simulink model "ThermalSystem2026 (3)"  (R2024b)
settings: Solver=VariableStepAuto  StartTime=0.0  StopTime=1296  RelTol=1e-3
settings Model: Creator=arthe  LastModifiedBy=arthe

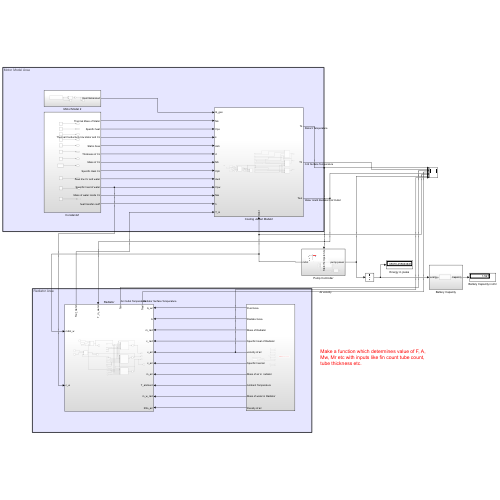
[thumbnail: Simulink's stored preview of the top-level diagram]
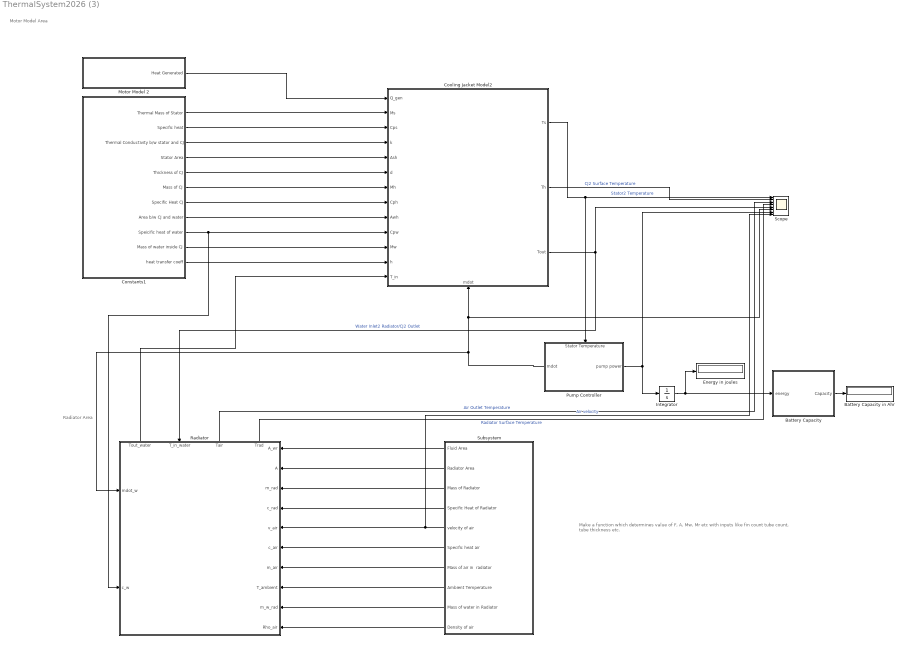
== system ThermalSystem2026 (3) ==
  note: Motor Model Area
  note: Radiator Area
  note: Make a function which determines value of F, A, Mw, Mr etc with inputs like fin count tube count, tube thickness etc.
  Battery Capacity : Subsystem
  Battery Capacity in Ahr : Display
  Constants1 : Subsystem
  Cooling Jacket Model2 : Subsystem
      settings: PortSchema="{\"entries\":[{\"content\":{\"sides\":[{\"content\":{\"connectorIds\":[\"In1\",\"In2\",\"In3\",\"In4\",\"In5\",\"In6\",\"In7\",\"In8\",\"In9\",\"In10\",\"In11\",\"In12\",\"In13\"]},\"type\":\"ConnectorPlacement.EquallySpacedRectSide\",\"uuid\":\"79d4d8e8-7803-45a2-afaa-4d22d6373157\"},{\"content\":{\"connectorIds\":[\"Out1\",\"Out2\",\"Out3\"],\"side\":\"RIGHT\"},\"type\":\"ConnectorPlacement.EquallySpacedRectSide\",\"uuid\":\"8eb2a985-3df9-4fca-ba99-d41949146ffd\"},{\"content\":{\"side\":\"TOP\"},\"type\":\"ConnectorPlacement.EquallySpacedRectSide\",\"uuid\":\"b6891a69-1971-4846-8973-0960fda02d22\"},{\"content\":{\"connectorIds\":[\"In14\"],\"side\":\"BOTTOM\"},\"type\":\"ConnectorPlacement.EquallySpacedRectSide\",\"uuid\":\"634c1221-39cf-4d03-a1b5-5507eb554710\"}]},\"type\":\"ConnectorPlacement.EquallySpacedConnector\",\"uuid\":\"d4f46766-14f9-4a8b-8c89-842668bdd4e0\"}],\"packageUris\":[\"http://schema.mathworks.com/mf0/Connector/R2020b\"],\"version\":\"1.0\"}"
  Energy in joules : Display
  Integrator : Integrator
  Motor Model 2 : Subsystem
  Pump Controller : Subsystem
      settings: PortSchema="{\"entries\":[{\"content\":{\"sides\":[{\"content\":{\"connectorIds\":[\"Out2\"]},\"type\":\"ConnectorPlacement.EquallySpacedRectSide\",\"uuid\":\"64509805-f0eb-407f-8df6-2012a67b9b8d\"},{\"content\":{\"connectorIds\":[\"Out1\"],\"side\":\"RIGHT\"},\"type\":\"ConnectorPlacement.EquallySpacedRectSide\",\"uuid\":\"85313de9-6d64-4d1e-8ebf-8c6fc6989453\"},{\"content\":{\"connectorIds\":[\"In1\"],\"side\":\"TOP\"},\"type\":\"ConnectorPlacement.EquallySpacedRectSide\",\"uuid\":\"4a1f9497-bef9-4f57-9d3c-2e3adca4de23\"}]},\"type\":\"ConnectorPlacement.EquallySpacedConnector\",\"uuid\":\"adca88aa-a89d-4531-9c32-6fc4488ac11c\"}],\"packageUris\":[\"http://schema.mathworks.com/mf0/Connector/R2020b\"],\"version\":\"1.0\"}"
  Radiator : Subsystem
      settings: PortSchema="{\"entries\":[{\"content\":{\"sides\":[{\"content\":{\"connectorIds\":[\"In1\",\"In2\",\"In3\",\"In4\",\"In5\",\"In6\",\"In7\",\"In8\",\"In9\",\"In10\"]},\"type\":\"ConnectorPlacement.EquallySpacedRectSide\",\"uuid\":\"442aa9ac-1748-45b5-b106-b2ea8ec9ba9a\"},{\"content\":{\"connectorIds\":[\"In12\",\"In13\"],\"side\":\"RIGHT\"},\"type\":\"ConnectorPlacement.EquallySpacedRectSide\",\"uuid\":\"346b8b1e-5690-410f-bffd-8882456125cf\"},{\"content\":{\"connectorIds\":[\"Out1\",\"Out2\",\"In11\",\"Out3\"],\"side\":\"TOP\"},\"type\":\"ConnectorPlacement.EquallySpacedRectSide\",\"uuid\":\"f47d136f-1f63-473a-b7aa-2f4bff6d0484\"}]},\"type\":\"ConnectorPlacement.EquallySpacedConnector\",\"uuid\":\"8ddbc53c-7178-458d-9bbd-f7e4bafa7e83\"}],\"packageUris\":[\"http://schema.mathworks.com/mf0/Connector/R2020b\"],\"version\":\"1.0\"}"
  Scope : Scope  NumInputPorts=8
  Subsystem : Subsystem
  wires:
  Constants1/7(Specific Heat CJ) -> Cooling Jacket Model2/8(Cph)
  Constants1/3(Thermal Conductivity b/w stator and CJ) -> Cooling Jacket Model2/4(k)
  Constants1/2(Specific heat) -> Cooling Jacket Model2/3(Cps)
  Constants1/11(heat transfer coeff) -> Cooling Jacket Model2/12(h)
  Constants1/10(Mass of water inside CJ) -> Cooling Jacket Model2/11(Mw)
  Constants1/8(Area b/w CJ and water) -> Cooling Jacket Model2/9(Awh)
  Constants1/5(Thickness of CJ) -> Cooling Jacket Model2/6(d)
  Constants1/1(Thermal Mass of Stator) -> Cooling Jacket Model2/2(Ms)
  Constants1/4(Stator Area) -> Cooling Jacket Model2/5(Ash)
  Constants1/6(Mass of CJ) -> Cooling Jacket Model2/7(Mh)
  Radiator/3(Tout_water) -> Cooling Jacket Model2/13(T_in)
  Cooling Jacket Model2/1(Ts) -> Scope/1, Pump Controller/1(Stator Temperature)  "Stator2 Temperature"
  Cooling Jacket Model2/2(Th) -> Scope/2  "CJ2 Surface Temperature"
  Cooling Jacket Model2/3(Tout) -> Radiator/11(T_in_water), Scope/5  "Water Inlet2 Radiator/CJ2 Outlet"
  Subsystem/8(Ambient Temperature) -> Radiator/8(T_ambient)
  Subsystem/3(Mass of Radiator) -> Radiator/3(m_rad)
  Subsystem/6(Specific heat air) -> Radiator/6(c_air)
  Subsystem/10(Density of air) -> Radiator/10(Rho_air)
  Subsystem/5(velocity of air) -> Scope/8, Radiator/5(v_air)  "Air velocity"
  Subsystem/4(Specific Heat of Radiator) -> Radiator/4(c_rad)
  Subsystem/7(Mass of air in  radiator) -> Radiator/7(m_air)
  Subsystem/9(Mass of water in Radiator) -> Radiator/9(m_w_rad)
  Subsystem/1("Fluid Area ") -> Radiator/1(A_wr)
  Subsystem/2(Radiator Area) -> Radiator/2(A)
  Radiator/1(Trad) -> Scope/4  "Radiator Surface Temperature"
  Radiator/2(Tair) -> Scope/3  "Air Outlet Temperature"
  Constants1/9(Speicific heat of water) -> Radiator/13(c_w), Cooling Jacket Model2/10(Cpw)
  Pump Controller/2(mdot) -> Radiator/12(mdot_w), Cooling Jacket Model2/14(mdot), Scope/6
  Pump Controller/1(pump power) -> Integrator/1, Scope/7
  Motor Model 2/1(Heat Generated) -> Cooling Jacket Model2/1(Q_gen)
  Integrator/1 -> Battery Capacity/1(energy), Energy in joules/1
  Battery Capacity/1(Capacity) -> Battery Capacity in Ahr/1

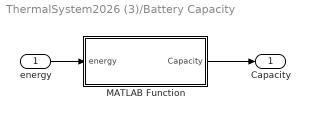
== system ThermalSystem2026 (3)/Battery Capacity ==
  energy : Inport
  MATLAB Function : MATLAB Function  TreatAsAtomicUnit=on
  Capacity : Outport
  wires:
  energy/1 -> MATLAB Function/1(energy)
  MATLAB Function/1(Capacity) -> Capacity/1

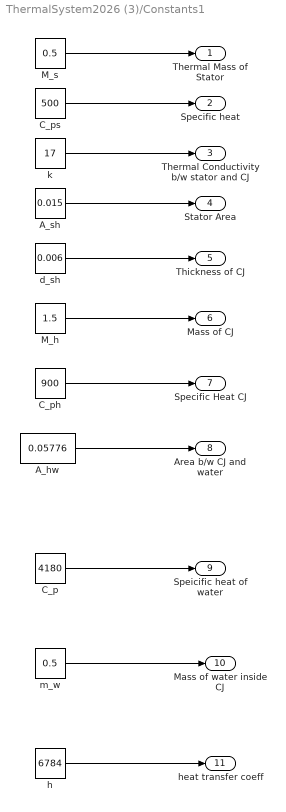
== system ThermalSystem2026 (3)/Constants1 ==
  A_hw : Constant  Value=0.05776
  A_sh : Constant  Value=0.015
  C_p : Constant  Value=4180
  C_ph : Constant  Value=900
  C_ps : Constant  Value=500
  M_h : Constant  Value=1.5
  M_s : Constant  Value=0.5
  d_sh : Constant  Value=0.006
  h : Constant  Value=6784
  k : Constant  Value=17
  m_w : Constant  Value=0.5
  Thermal Mass of Stator : Outport
  Specific heat : Outport  Port=2
  Thermal Conductivity b/w stator and CJ : Outport  Port=3
  Stator Area : Outport  Port=4
  Thickness of CJ : Outport  Port=5
  Mass of CJ : Outport  Port=6
  Specific Heat CJ : Outport  Port=7
  Area b/w CJ and water : Outport  Port=8
  Speicific heat of water : Outport  Port=9
  Mass of water inside CJ : Outport  Port=10
  heat transfer coeff : Outport  Port=11
  wires:
  C_ph/1 -> Specific Heat CJ/1
  A_sh/1 -> Stator Area/1
  C_ps/1 -> Specific heat/1
  M_s/1 -> Thermal Mass of Stator/1
  d_sh/1 -> Thickness of CJ/1
  m_w/1 -> Mass of water inside CJ/1
  k/1 -> Thermal Conductivity b/w stator and CJ/1
  M_h/1 -> Mass of CJ/1
  A_hw/1 -> Area b/w CJ and water/1
  C_p/1 -> Speicific heat of water/1
  h/1 -> heat transfer coeff/1

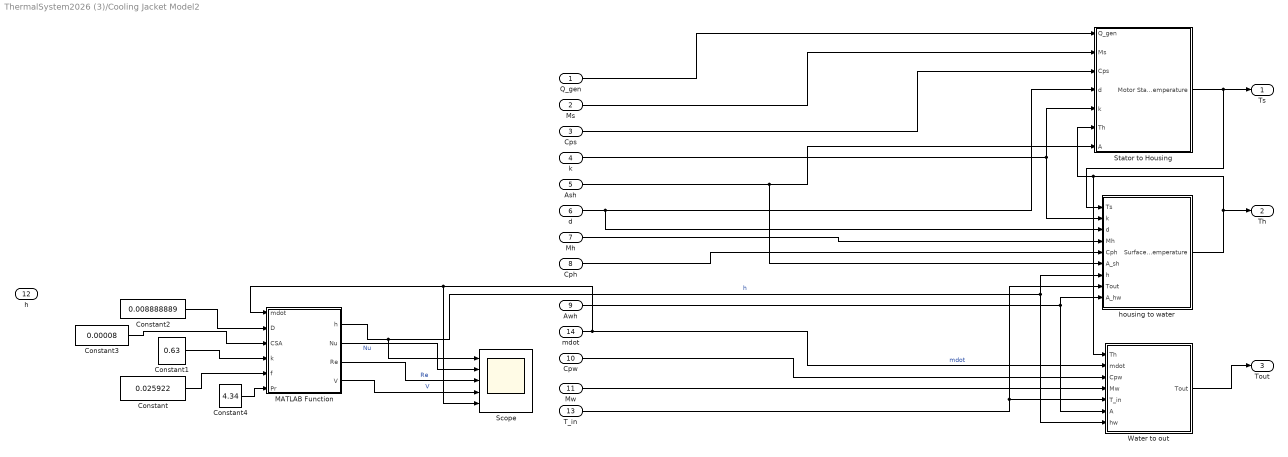
== system ThermalSystem2026 (3)/Cooling Jacket Model2 ==
  Q_gen : Inport
  Ms : Inport  Port=2
  Cps : Inport  Port=3
  k : Inport  Port=4
  Ash : Inport  Port=5
  d : Inport  Port=6
  Mh : Inport  Port=7
  Cph : Inport  Port=8
  Awh : Inport  Port=9
  Cpw : Inport  Port=10
  Mw : Inport  Port=11
  h : Inport  Port=12
  T_in : Inport  Port=13
  mdot : Inport  Port=14
  Constant : Constant  Value=0.025922
  Constant1 : Constant  Value=0.63
  Constant2 : Constant  Value=0.008888889
  Constant3 : Constant  Value=0.00008
  Constant4 : Constant  Value=4.34
  MATLAB Function : MATLAB Function  TreatAsAtomicUnit=on
  Scope : Scope  NumInputPorts=5
  Stator to Housing : Subsystem
  Water to out : Subsystem
  housing to water : Subsystem
  Ts : Outport
  Th : Outport  Port=2
  Tout : Outport  Port=3
  wires:
  mdot/1 -> MATLAB Function/1(mdot), Scope/5, Water to out/2(mdot)  "mdot"
  Stator to Housing/1(Motor Stator Temperature) -> Ts/1, housing to water/1(Ts)
  Water to out/1(Tout) -> Tout/1
  housing to water/1(Surface Temperature) -> Stator to Housing/6(Th), Water to out/1(Th), Th/1
  d/1 -> housing to water/3(d), Stator to Housing/4(d)
  Cpw/1 -> Water to out/3(Cpw)
  Mw/1 -> Water to out/4(Mw)
  Q_gen/1 -> Stator to Housing/1(Q_gen)
  Ms/1 -> Stator to Housing/2(Ms)
  Cps/1 -> Stator to Housing/3(Cps)
  Ash/1 -> housing to water/6(A_sh), Stator to Housing/7(A)
  T_in/1 -> housing to water/8(Tout), Water to out/5(T_in)
  Mh/1 -> housing to water/4(Mh)
  Cph/1 -> housing to water/5(Cph)
  k/1 -> housing to water/2(k), Stator to Housing/5(k)
  MATLAB Function/1(h) -> Scope/1, housing to water/7(h), Water to out/7(hw)  "h"
  Awh/1 -> housing to water/9(A_hw), Water to out/6(A)
  Constant/1 -> MATLAB Function/5(f)
  Constant1/1 -> MATLAB Function/4(k)
  Constant2/1 -> MATLAB Function/2(D)
  Constant3/1 -> MATLAB Function/3(CSA)
  Constant4/1 -> MATLAB Function/6(Pr)
  MATLAB Function/2(Nu) -> Scope/2  "Nu"
  MATLAB Function/3(Re) -> Scope/3  "Re"
  MATLAB Function/4(V) -> Scope/4  "V"

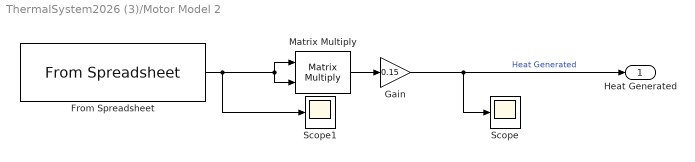
== system ThermalSystem2026 (3)/Motor Model 2 ==
  From Spreadsheet : FromSpreadsheet  FileName=expanded_data.xlsx  SampleTime=1
  Gain : Gain  Gain=0.15
  Matrix Multiply : Product  Multiplication=Matrix(*)
  Scope : Scope
  Scope1 : Scope
  Heat Generated : Outport
  wires:
  Matrix Multiply/1 -> Gain/1
  From Spreadsheet/1 -> Scope1/1, Matrix Multiply/2, Matrix Multiply/1
  Gain/1 -> Scope/1, Heat Generated/1  "Heat Generated"

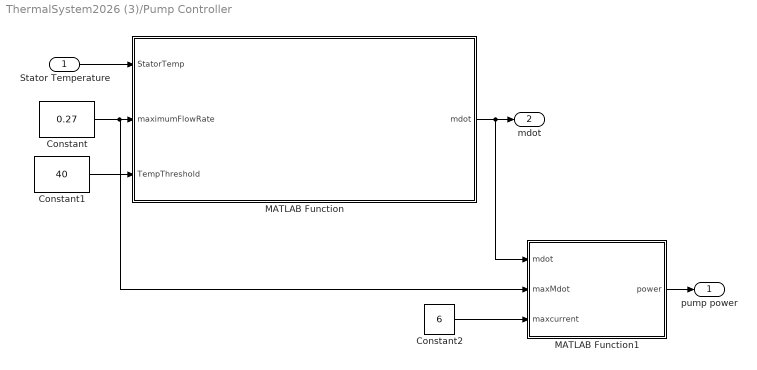
== system ThermalSystem2026 (3)/Pump Controller ==
  Stator Temperature : Inport
  Constant : Constant  Value=0.27
  Constant1 : Constant  Value=40
  Constant2 : Constant  Value=6
  MATLAB Function : MATLAB Function  TreatAsAtomicUnit=on
  MATLAB Function1 : MATLAB Function  TreatAsAtomicUnit=on
  pump power : Outport
  mdot : Outport  Port=2
  wires:
  Constant/1 -> MATLAB Function1/2(maxMdot), MATLAB Function/2(maximumFlowRate)
  MATLAB Function/1(mdot) -> MATLAB Function1/1(mdot), mdot/1
  Stator Temperature/1 -> MATLAB Function/1(StatorTemp)
  Constant1/1 -> MATLAB Function/3(TempThreshold)
  Constant2/1 -> MATLAB Function1/3(maxcurrent)
  MATLAB Function1/1(power) -> pump power/1

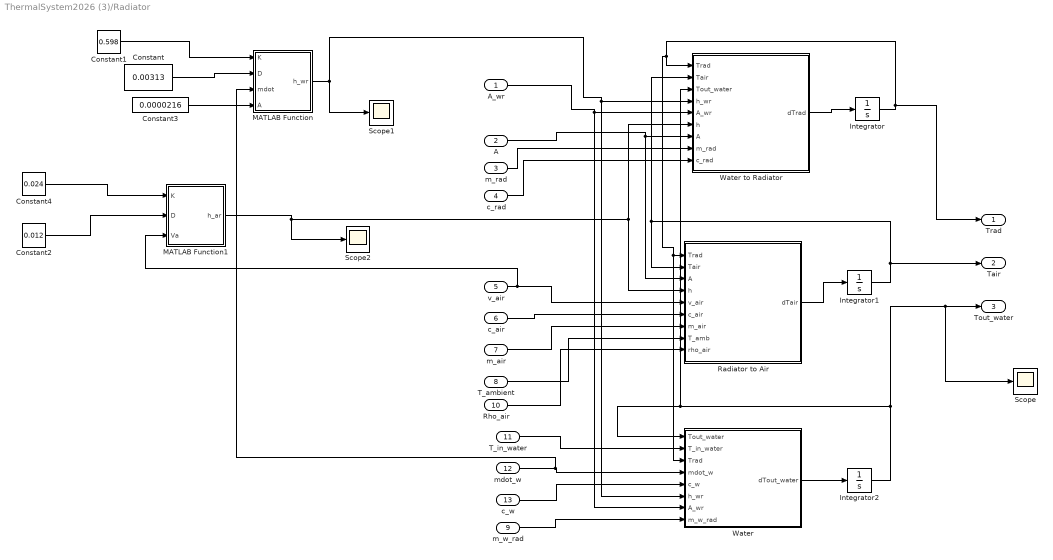
== system ThermalSystem2026 (3)/Radiator ==
  A_wr : Inport
  A : Inport  Port=2
  m_rad : Inport  Port=3
  c_rad : Inport  Port=4
  v_air : Inport  Port=5
  c_air : Inport  Port=6
  m_air : Inport  Port=7
  T_ambient : Inport  Port=8
  m_w_rad : Inport  Port=9
  Rho_air : Inport  Port=10
  T_in_water : Inport  Port=11
  mdot_w : Inport  Port=12
  c_w : Inport  Port=13
  Constant : Constant  Value=0.00313
  Constant1 : Constant  Value=0.598
  Constant2 : Constant  Value=0.012
  Constant3 : Constant  Value=0.0000216
  Constant4 : Constant  Value=0.024
  Integrator : Integrator  InitialCondition=35
  Integrator1 : Integrator  InitialCondition=35
  Integrator2 : Integrator  InitialCondition=35
  MATLAB Function : MATLAB Function  TreatAsAtomicUnit=on
  MATLAB Function1 : MATLAB Function  TreatAsAtomicUnit=on
  Radiator to Air : MATLAB Function  TreatAsAtomicUnit=on
  Scope : Scope
  Scope1 : Scope
  Scope2 : Scope
  Water : MATLAB Function  TreatAsAtomicUnit=on
  Water to Radiator : MATLAB Function  TreatAsAtomicUnit=on
  Trad : Outport
  Tair : Outport  Port=2
  Tout_water : Outport  Port=3
  wires:
  Water/1(dTout_water) -> Integrator2/1
  Integrator2/1 -> Scope/1, Tout_water/1, Water/1(Tout_water), Water to Radiator/3(Tout_water)
  Radiator to Air/1(dTair) -> Integrator1/1
  Water to Radiator/1(dTrad) -> Integrator/1
  MATLAB Function/1(h_wr) -> Scope1/1, Water/6(h_wr), Water to Radiator/4(h_wr)
  A_wr/1 -> Water/7(A_wr), Water to Radiator/5(A_wr)
  A/1 -> Radiator to Air/3(A), Water to Radiator/7(A)
  MATLAB Function1/1(h_ar) -> Water to Radiator/6(h), Radiator to Air/4(h), Scope2/1
  m_rad/1 -> Water to Radiator/8(m_rad)
  c_rad/1 -> Water to Radiator/9(c_rad)
  c_air/1 -> Radiator to Air/6(c_air)
  m_air/1 -> Radiator to Air/7(m_air)
  T_ambient/1 -> Radiator to Air/8(T_amb)
  Integrator1/1 -> Radiator to Air/2(Tair), Water to Radiator/2(Tair), Tair/1
  c_w/1 -> Water/5(c_w)
  m_w_rad/1 -> Water/8(m_w_rad)
  T_in_water/1 -> Water/2(T_in_water)
  Integrator/1 -> Water/3(Trad), Radiator to Air/1(Trad), Water to Radiator/1(Trad), Trad/1
  mdot_w/1 -> MATLAB Function/3(mdot), Water/4(mdot_w)
  Rho_air/1 -> Radiator to Air/9(rho_air)
  Constant/1 -> MATLAB Function/2(D)
  Constant1/1 -> MATLAB Function/1(K)
  Constant3/1 -> MATLAB Function/4(A)
  Constant4/1 -> MATLAB Function1/1(K)
  Constant2/1 -> MATLAB Function1/2(D)
  v_air/1 -> MATLAB Function1/3(Va), Radiator to Air/5(v_air)

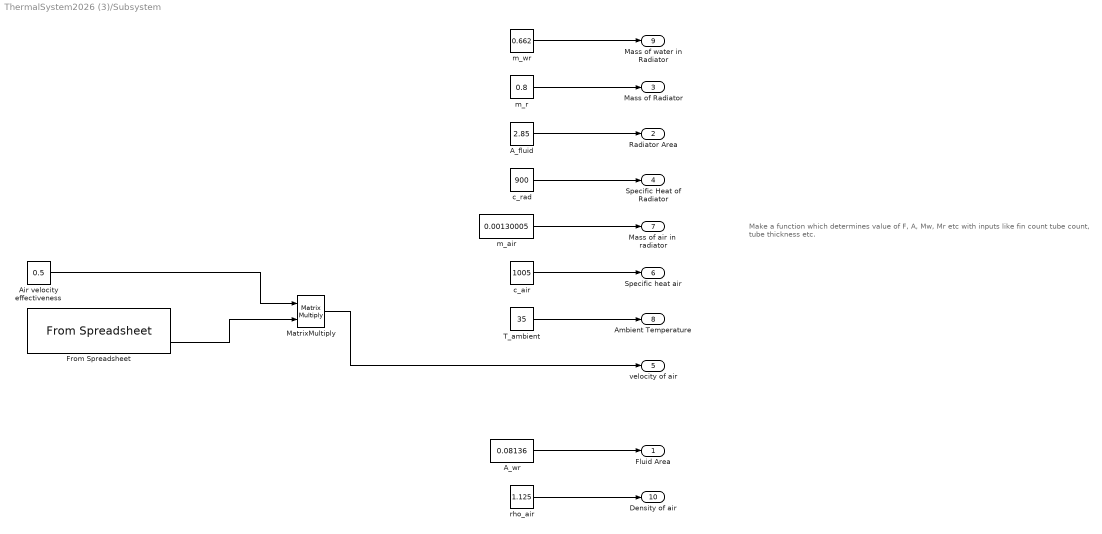
== system ThermalSystem2026 (3)/Subsystem ==
  note: Make a function which determines value of F, A, Mw, Mr etc with inputs like fin count tube count, tube thickness etc.
  A_fluid : Constant  Value=2.85
  A_wr : Constant  Value=0.08136
  Air velocity effectiveness : Constant  Value=0.5
  From Spreadsheet : FromSpreadsheet  FileName=speedvstimefiltered.xlsx  SampleTime=1
  MatrixMultiply : Product  Multiplication=Matrix(*)
  T_ambient : Constant  Value=35
  c_air : Constant  Value=1005
  c_rad : Constant  Value=900
  m_air : Constant  Value=0.00130005
  m_r : Constant  Value=0.8
  m_wr : Constant  Value=0.662
  rho_air : Constant  Value=1.125
  "Fluid Area " : Outport
  Radiator Area : Outport  Port=2
  Mass of Radiator : Outport  Port=3
  Specific Heat of Radiator : Outport  Port=4
  velocity of air : Outport  Port=5
  Specific heat air : Outport  Port=6
  Mass of air in  radiator : Outport  Port=7
  Ambient Temperature : Outport  Port=8
  Mass of water in Radiator : Outport  Port=9
  Density of air : Outport  Port=10
  wires:
  A_fluid/1 -> Radiator Area/1
  T_ambient/1 -> Ambient Temperature/1
  m_wr/1 -> Mass of water in Radiator/1
  MatrixMultiply/1 -> velocity of air/1
  c_rad/1 -> Specific Heat of Radiator/1
  m_r/1 -> Mass of Radiator/1
  A_wr/1 -> "Fluid Area "/1
  rho_air/1 -> Density of air/1
  m_air/1 -> Mass of air in  radiator/1
  c_air/1 -> Specific heat air/1
  From Spreadsheet/2 -> MatrixMultiply/2
  Air velocity effectiveness/1 -> MatrixMultiply/1

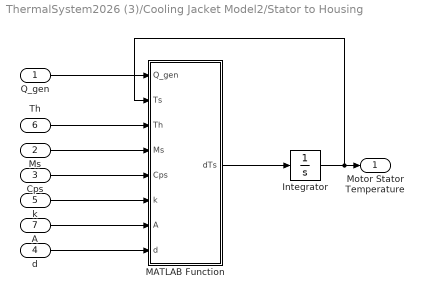
== system ThermalSystem2026 (3)/Cooling Jacket Model2/Stator to Housing ==
  Q_gen : Inport
  Ms : Inport  Port=2
  Cps : Inport  Port=3
  d : Inport  Port=4
  k : Inport  Port=5
  Th : Inport  Port=6
  A : Inport  Port=7
  Integrator : Integrator  InitialCondition=35
  MATLAB Function : MATLAB Function  TreatAsAtomicUnit=on
  Motor Stator Temperature : Outport
  wires:
  MATLAB Function/1(dTs) -> Integrator/1
  Cps/1 -> MATLAB Function/5(Cps)
  k/1 -> MATLAB Function/6(k)
  Ms/1 -> MATLAB Function/4(Ms)
  d/1 -> MATLAB Function/8(d)
  A/1 -> MATLAB Function/7(A)
  Q_gen/1 -> MATLAB Function/1(Q_gen)
  Integrator/1 -> MATLAB Function/2(Ts), Motor Stator Temperature/1
  Th/1 -> MATLAB Function/3(Th)

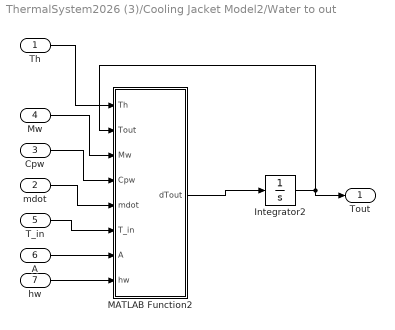
== system ThermalSystem2026 (3)/Cooling Jacket Model2/Water to out ==
  Th : Inport
  mdot : Inport  Port=2
  Cpw : Inport  Port=3
  Mw : Inport  Port=4
  T_in : Inport  Port=5
  A : Inport  Port=6
  hw : Inport  Port=7
  Integrator2 : Integrator  InitialCondition=35
  MATLAB Function2 : MATLAB Function  TreatAsAtomicUnit=on
  Tout : Outport
  wires:
  Integrator2/1 -> Tout/1, MATLAB Function2/2(Tout)
  MATLAB Function2/1(dTout) -> Integrator2/1
  Th/1 -> MATLAB Function2/1(Th)
  T_in/1 -> MATLAB Function2/6(T_in)
  Mw/1 -> MATLAB Function2/3(Mw)
  mdot/1 -> MATLAB Function2/5(mdot)
  Cpw/1 -> MATLAB Function2/4(Cpw)
  A/1 -> MATLAB Function2/7(A)
  hw/1 -> MATLAB Function2/8(hw)

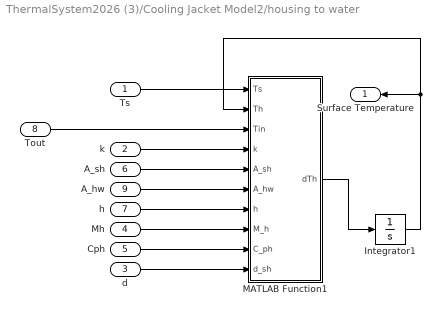
== system ThermalSystem2026 (3)/Cooling Jacket Model2/housing to water ==
  Ts : Inport
  k : Inport  Port=2
  d : Inport  Port=3
  Mh : Inport  Port=4
  Cph : Inport  Port=5
  A_sh : Inport  Port=6
  h : Inport  Port=7
  Tout : Inport  Port=8
  A_hw : Inport  Port=9
  Integrator1 : Integrator  InitialCondition=35
  MATLAB Function1 : MATLAB Function  TreatAsAtomicUnit=on
  Surface Temperature : Outport
  wires:
  MATLAB Function1/1(dTh) -> Integrator1/1
  k/1 -> MATLAB Function1/4(k)
  Ts/1 -> MATLAB Function1/1(Ts)
  Tout/1 -> MATLAB Function1/3(Tin)
  Integrator1/1 -> MATLAB Function1/2(Th), Surface Temperature/1
  d/1 -> MATLAB Function1/10(d_sh)
  Cph/1 -> MATLAB Function1/9(C_ph)
  Mh/1 -> MATLAB Function1/8(M_h)
  A_hw/1 -> MATLAB Function1/6(A_hw)
  A_sh/1 -> MATLAB Function1/5(A_sh)
  h/1 -> MATLAB Function1/7(h)

== matlab function ThermalSystem2026 (3)/Radiator/MATLAB Function1 ==
  data: K input; h_ar output; D input; Va input
function h_ar = fcn(K, D, Va)
Nu = 0.664*((Va*D)/0.0000148)^0.5*(0.71)^0.33;
h_ar = (Nu * K)/D;
end

== matlab function ThermalSystem2026 (3)/Cooling Jacket Model2/MATLAB Function ==
  data: mdot input; h output; D input; CSA input; k input; f input; Pr input; Nu output; Re output; V output
function [h, Nu, Re, V]= fcn(mdot, D, CSA, k, f, Pr)
V = mdot/(1000*CSA);
Re = (V*1000*D)/0.00089;
Nu = ((f/8)*(Re-1000)*Pr)/(1+(12.7*(f/8)^0.5 * (Pr^(2/3) - 1)));
h = (Nu*k)/D;
end

== matlab function ThermalSystem2026 (3)/Battery Capacity/MATLAB Function ==
  data: Capacity output; energy input
function Capacity = fcn(energy)
    Capacity = energy/(12*3600);
end

== matlab function ThermalSystem2026 (3)/Cooling Jacket Model2/Stator to Housing/MATLAB Function ==
  data: Q_gen input; Ts input; dTs output; Th input; Ms input; Cps input; k input; A input; d input
function dTs = f1(Q_gen, Ts, Th, Ms, Cps, k, A, d)
    dTs = (Q_gen - (Ts - Th) * k * A / d) / (Ms * Cps);
end

== matlab function ThermalSystem2026 (3)/Cooling Jacket Model2/Water to out/MATLAB Function2 ==
  data: Th input; Tout input; Mw input; Cpw input; mdot input; T_in input; dTout output; A input; hw input
function dTout = f3(Th, Tout, Mw, Cpw, mdot, T_in, A, hw)
    q_from_housing = (Th - Tout) * hw * A;
    q_out = (Tout - T_in) * mdot * Cpw;
    dTout = ((q_from_housing - q_out)) / (Mw * Cpw);
end

== matlab function ThermalSystem2026 (3)/Cooling Jacket Model2/housing to water/MATLAB Function1 ==
  data: Ts input; Th input; Tin input; k input; A_sh input; A_hw input; dTh output; h input; M_h input; C_ph input; d_sh input
function dTh = f2(Ts, Th, Tin, k, A_sh, A_hw, h, M_h, C_ph, d_sh)
    dTh = ((k*A_sh*(Ts - Th)/d_sh) - h*A_hw*(Th - Tin)) / (M_h * C_ph);
end

== matlab function ThermalSystem2026 (3)/Pump Controller/MATLAB Function1 ==
  data: mdot input; power output; maxMdot input; maxcurrent input
function power = fcn(mdot, maxMdot, maxcurrent)
    power = (((4-maxcurrent)/(0-maxMdot))*(mdot - maxMdot) + maxcurrent)*12;
end

== matlab function ThermalSystem2026 (3)/Pump Controller/MATLAB Function ==
  data: StatorTemp input; mdot output; maximumFlowRate input; TempThreshold input
function mdot = fcn(StatorTemp, maximumFlowRate, TempThreshold)
if StatorTemp < 80 && StatorTemp > TempThreshold
    mdot = ((StatorTemp-TempThreshold)/(80 - TempThreshold))*maximumFlowRate;
elseif StatorTemp < TempThreshold
    mdot = 0;
else
    mdot = maximumFlowRate;
end
end

== matlab function ThermalSystem2026 (3)/Radiator/MATLAB Function ==
  data: K input; h_wr output; D input; mdot input; A input
function h_wr = fcn(K, D, mdot, A)
Vm = mdot/(A * 24 * 1000);
Nu = 0.023 * (((1000*D*Vm)/0.001002)^0.8) * (6.9^0.4);
h_wr = (Nu * K)/D;
end

== matlab function ThermalSystem2026 (3)/Radiator/Water to Radiator ==
  data: Trad input; Tair input; dTrad output; Tout_water input; h_wr input; A_wr input; h input; A input; m_rad input; c_rad input
function dTrad = f1(Trad, Tair, Tout_water, h_wr, A_wr, h, A, m_rad, c_rad)
    dTrad = ((Tout_water - Trad) * h_wr * A_wr - (Trad - Tair) * h * A) / (m_rad * c_rad);
end

== matlab function ThermalSystem2026 (3)/Radiator/Radiator to Air ==
  data: Trad input; Tair input; dTair output; A input; h input; v_air input; c_air input; m_air input; T_amb input; rho_air input
function dTair = f2(Trad, Tair, A, h, v_air, c_air, m_air, T_amb, rho_air)
    dTair = ((Trad - Tair) * h * A - (Tair - T_amb) * v_air * rho_air * A * c_air) / (m_air * c_air);
end

== matlab function ThermalSystem2026 (3)/Radiator/Water ==
  data: Tout_water input; T_in_water input; Trad input; dTout_water output; mdot_w input; c_w input; h_wr input; A_wr input; m_w_rad input
function dTout_water = f3(Tout_water, T_in_water, Trad, mdot_w, c_w, h_wr, A_wr, m_w_rad)
    dTout_water = ((T_in_water - Tout_water) * mdot_w * c_w - (Tout_water - Trad) * h_wr * A_wr) / (m_w_rad * c_w);
end
